simulink model "simulacaoMaquinaCC"  (R2022a)
settings: Solver=VariableStepAuto  StartTime=0.0  StopTime=0.5  RelTol=1e-3
libraries: spsDCVoltageSourceLib x2, spsCurrentMeasurementLib x1, spsDCMachineLib x1, spspowerguiLib x1
settings Model: Creator=marcone.faria  LastModifiedBy=marcone.faria

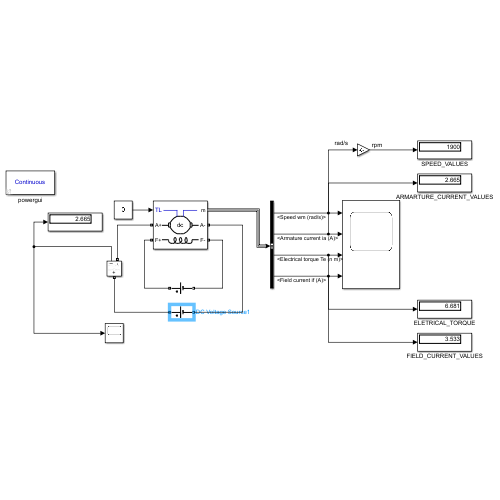
[thumbnail: Simulink's stored preview of the top-level diagram]
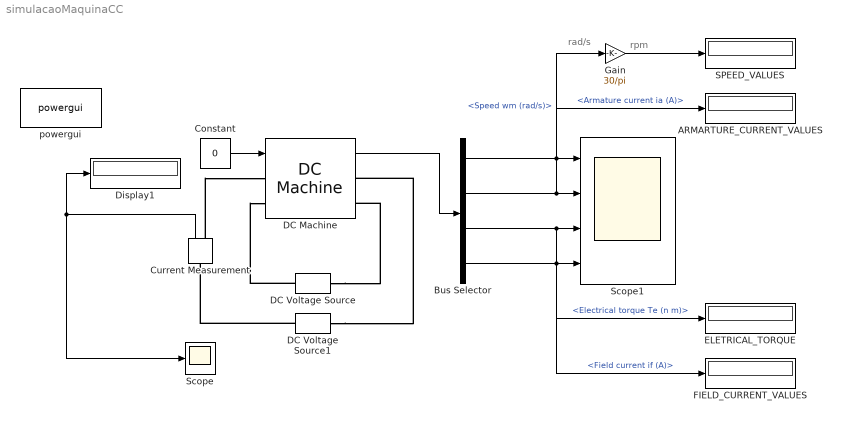
== system simulacaoMaquinaCC ==
  note: rad/s
  note: rpm
  ARMARTURE_CURRENT_VALUES : Display
  Bus Selector : BusSelector  OutputSignals=Speed wm (rad/s),Armature current ia (A),Electrical torque Te (n m),Field current if (A)
  Constant : Constant  Value=0
  Current Measurement : spsCurrentMeasurementLib/Current Measurement  PhasorSimulation=off  OutputType=Complex  PSBequivalent=0
  DC Machine : spsDCMachineLib/DC Machine  PresetModel=04: 10HP 240V 1750RPM Field:300V  MechanicalLoad=Torque TL  FieldType=Wound  ShowDetailedParameters=on  MeasurementBus=off  RLa=[1.086 0.01216]  RLf=[180 71.47]  Laf=0.6458  MachineConstant=Torque constant (N.m/A)  Ke=1.8  Kt=1.8  J=0.04251  Bm=0.003406  Tf=1.046  w0=1  Ifinit=3.53315274997056  TsPowergui=0  TsBlock=-1
  DC Voltage Source : spsDCVoltageSourceLib/DC Voltage Source  Amplitude=300  Measurements=None
  DC Voltage Source1 : spsDCVoltageSourceLib/DC Voltage Source  Amplitude=240  Measurements=None
  Display1 : Display
  ELETRICAL_TORQUE : Display
  FIELD_CURRENT_VALUES : Display
  Gain : Gain  Gain=30/pi
  SPEED_VALUES : Display
  Scope : Scope
  Scope1 : Scope  NumInputPorts=4
  powergui : spspowerguiLib/powergui  Priority=1  SimulationMode=Continuous  SampleTime=50e-6  frequency=60  Iterations=50  frequencyindice=0  Pbase=100e6  ErrMax=1e-4  UnitsV=kV  UnitsW=MW  buscounter=0  FunctionMessages=off  echomessages=off  EnableUseOfTLC=off  CurrentSourceSwitches=off  DisableSnubberDevices=off  DisableRonSwitches=off  DisableVfSwitches=off  DisplayEquations=off  AutomaticDiscreteSolvers=off  SolverType=Tustin/Backward Euler (TBE)  Interpol=off  ExternalGateDelay=off  methode=off  Ts=100  x0status=blocks  SPID=on  SwTol=0  HookPort=off  NonlinearTolerance=1e-4  nMaxIteration=100  ContinueOnMaxIteration=off  RestoreLinks=warning  ResistiveCurrentMeasurement=off  Frange=[0:2:500]  Ylog=off  Xlog=on  ShowGrid=off  save=off  variable=ZData  structure=0  ZoomFFT=off  StartTime=0.0  cycles=1  DisplayStyle=1  fundamental=60  FreqAxis=off  MaxFrequency=1000  frequencyindicesteady=1  RmsSteady=1  display=off
  wires:
  Current Measurement/1 -> Scope/1, Display1/1
  DC Machine/1 -> Bus Selector/1
  Constant/1 -> DC Machine/1
  Bus Selector/1 -> Scope1/1, Gain/1  "<Speed wm (rad/s)>"
  Bus Selector/2 -> ARMARTURE_CURRENT_VALUES/1, Scope1/2  "<Armature current ia (A)>"
  Bus Selector/3 -> Scope1/3, ELETRICAL_TORQUE/1  "<Electrical torque Te (n m)>"
  Bus Selector/4 -> Scope1/4, FIELD_CURRENT_VALUES/1  "<Field current if (A)>"
  Gain/1 -> SPEED_VALUES/1
  connections:
  DC Voltage Source/RConn1 -- DC Machine/LConn2
  DC Voltage Source/LConn1 -- DC Machine/RConn2
  DC Voltage Source1/RConn1 -- Current Measurement/LConn1
  DC Voltage Source1/LConn1 -- DC Machine/RConn1
  Current Measurement/RConn1 -- DC Machine/LConn1
